simulink model "Consensus_Swarm"  (R2023b)
settings: Solver=ode3  StartTime=0.0  StopTime=inf  FixedStep=0.001  RelTol=1e-3
values from neighbouring files (symbols this model uses):
  g = 9.8    [Parameters.m]
  Ic = [2 0 0; 0 2 0; 0 0 4]    [Parameters.m]
  m = 1    [Parameters.m]
  M_RB = [eye(3), zeros(3); zeros(3), I]    [Parameters.m]
  SAVE_SPACE = 5    [Parameters.m]
  STEP_SIZE = 1    [Parameters.m]
libraries: simulink_extras x36, slpidlib x36, aerolibutil x12, vrlib x7
(part 2 of 6)

== system Consensus_Swarm/Formatting/Euler to VR5 ==
  Euler Angles : Inport
  Axis Angle Vector : Subsystem
  Mux : Mux  Inputs=2
  Mux1 : Mux  Inputs=2
  Mux2 : Mux  Inputs=2
  Quaternion Multiplication (Pitch & Yaw) : aerolibutil/Quaternion Multiplication
  Quaternion Multiplication (Roll) : aerolibutil/Quaternion Multiplication
  Quaternion Normalization : Subsystem
  Quaternion Normalization1 : Subsystem
  Quaternion Normalization2 : Subsystem
  Selector : Selector  InputPortWidth=3  IndexOptions=Index vector (dialog)  Indices=[3]  OutputSizes=1
  Selector1 : Selector  InputPortWidth=3  IndexOptions=Index vector (dialog)  Indices=[2]  OutputSizes=1
  Selector2 : Selector  InputPortWidth=3  IndexOptions=Index vector (dialog)  Indices=[1]  OutputSizes=1
  Vr Pitch Axes : Constant  Value=[0 0 1]
  Vr Roll Axes : Constant  Value=[1 0 0]
  Vr Yaw Axes : Constant  Value=[0 -1 0]
  Axis Angle : Outport  VectorParamsAs1DForOutWhenUnconnected=off
  wires:
  Quaternion Multiplication (Roll)/1 -> Axis Angle Vector/1(e0)
  Axis Angle Vector/1(e0_norm) -> Axis Angle/1
  Quaternion Normalization/1(e0_norm) -> Quaternion Multiplication (Roll)/2
  Quaternion Normalization2/1(e0_norm) -> Quaternion Multiplication (Pitch & Yaw)/1
  Quaternion Normalization1/1(e0_norm) -> Quaternion Multiplication (Pitch & Yaw)/2
  Mux2/1 -> Quaternion Normalization2/1(e0)
  Mux1/1 -> Quaternion Normalization1/1(e0)
  Mux/1 -> Quaternion Normalization/1(e0)
  Selector/1 -> Mux2/1
  Vr Yaw Axes/1 -> Mux2/2
  Selector1/1 -> Mux1/1
  Vr Pitch Axes/1 -> Mux1/2
  Selector2/1 -> Mux/1
  Vr Roll Axes/1 -> Mux/2
  Euler Angles/1 -> Selector2/1, Selector1/1, Selector/1
  Quaternion Multiplication (Pitch & Yaw)/1 -> Quaternion Multiplication (Roll)/1

== system Consensus_Swarm/Formatting/Subsystem ==
  Propeller velocities : Inport
  Bias : Bias  Bias=.1  SaturateOnIntegerOverflow=off
  Bias1 : Bias  Bias=-.3  SaturateOnIntegerOverflow=off
  Bias2 : Bias  Bias=.5  SaturateOnIntegerOverflow=off
  Bias3 : Bias  Bias=.7  SaturateOnIntegerOverflow=off
  Constant : Constant  Value=[0 1 0]
  Data Type Conversion : DataTypeConversion  OutDataTypeStr=double  SaturateOnIntegerOverflow=off  RndMeth=Floor
  Demux : Demux
  Gain : Gain  Gain=1.38408
  Integrator : Integrator  InitialCondition=[.1 ; .2 ;-.3 ;-.4]  WrapState=on  WrappedStateUpperValue=2*pi  WrappedStateLowerValue=-2*pi
  Mux{,1..3} (4 alike) : Mux  Inputs=2
  Rate Transition2 : RateTransition
  Position Blade1 : Outport  VectorParamsAs1DForOutWhenUnconnected=off
  Position Blade 2 : Outport  Port=2  VectorParamsAs1DForOutWhenUnconnected=off
  Position Blade 3 : Outport  Port=3  VectorParamsAs1DForOutWhenUnconnected=off
  Position Blade 4 : Outport  Port=4  VectorParamsAs1DForOutWhenUnconnected=off
  wires:
  Bias3/1 -> Mux3/2
  Mux3/1 -> Position Blade 4/1
  Bias1/1 -> Mux1/2
  Bias2/1 -> Mux2/2
  Demux/2 -> Bias1/1
  Constant/1 -> Mux3/1, Mux2/1, Mux1/1, Mux/1
  Mux1/1 -> Position Blade 2/1
  Mux2/1 -> Position Blade 3/1
  Integrator/1 -> Rate Transition2/1
  Mux/1 -> Position Blade1/1
  Demux/3 -> Bias2/1
  Bias/1 -> Mux/2
  Propeller velocities/1 -> Data Type Conversion/1
  Demux/4 -> Bias3/1
  Rate Transition2/1 -> Demux/1
  Demux/1 -> Bias/1
  Data Type Conversion/1 -> Gain/1
  Gain/1 -> Integrator/1

== system Consensus_Swarm/Subsystem/LIDER ==
  (x,y,z,psi) : Inport
  GamePad : Inport  Port=2
  Constant2 : Constant  Value=[0;-0;-40]  VectorParams1D=off
  Degrees to Radians : simulink_extras/Transformations/Degrees to Radians
  Demux1 : Demux  Outputs=6
  Flight Control System : Subsystem
      settings: PortSchema="{\"entries\":[{\"content\":{\"sides\":[{\"content\":{\"connectorIds\":[\"In1\",\"In2\"]},\"type\":\"ConnectorPlacement.EquallySpacedRectSide\",\"uuid\":\"8ffec179-99fb-4b4c-a09d-a73fa0154dea\"},{\"content\":{\"connectorIds\":[\"Out1\"],\"side\":\"RIGHT\"},\"type\":\"ConnectorPlacement.EquallySpacedRectSide\",\"uuid\":\"b9ff487d-1da1-449a-81c9-f1838b0d3727\"},{\"content\":{\"connectorIds\":[\"In3\"],\"side\":\"TOP\"},\"type\":\"ConnectorPlacement.EquallySpacedRectSide\",\"uuid\":\"1948ac9a-8b1f-4a62-833b-18e2b106d39d\"}]},\"type\":\"ConnectorPlacement.EquallySpacedConnector\",\"uuid\":\"fea635f7-9753-4696-bad7-e2485c1b5acc\"}],\"packageUris\":[\"http://schema.mathworks.com/mf0/Connector/R2020b\"],\"version\":\"1.0\"}"
  Manual Switch : ManualSwitch  CurrentSetting=0
  Manual Switch1 : ManualSwitch  CurrentSetting=0
  Mux : Mux  Inputs=2
  OL inputs : Constant  Value=[0;0;0;0]  VectorParams1D=off
  Position refs (x,y,z,psi) : Constant  Value=[20;20;-17;-45]  VectorParams1D=off
  Quadcopter model : Subsystem
      settings: PortSchema="{\"entries\":[{\"content\":{\"sides\":[{\"content\":{\"connectorIds\":[\"In1\"]},\"type\":\"ConnectorPlacement.EquallySpacedRectSide\",\"uuid\":\"c5c2dfb8-9ff8-4aa4-96a6-7fa0d886c51f\"},{\"content\":{\"connectorIds\":[\"Out1\"],\"side\":\"RIGHT\"},\"type\":\"ConnectorPlacement.EquallySpacedRectSide\",\"uuid\":\"2d7c7d5c-4ac5-4ebd-b09f-6a78733e851d\"},{\"content\":{\"connectorIds\":[\"In2\"],\"side\":\"TOP\"},\"type\":\"ConnectorPlacement.EquallySpacedRectSide\",\"uuid\":\"cf3a786d-06ed-46d4-985b-5c210afb13ec\"}]},\"type\":\"ConnectorPlacement.EquallySpacedConnector\",\"uuid\":\"cd57f0e6-7b9c-4392-8478-6e8af8e2560e\"}],\"packageUris\":[\"http://schema.mathworks.com/mf0/Connector/R2020b\"],\"version\":\"1.0\"}"
  Radians to Degrees : simulink_extras/Transformations/Radians to Degrees
  Radians to Degrees1 : simulink_extras/Transformations/Radians to Degrees
  Radians to Degrees2 : simulink_extras/Transformations/Radians to Degrees
  p(0) : Constant  Value=[100;100;-100]  VectorParams1D=off
  phi(t) : Scope
  psi(t) : Scope
  theta(t) : Scope
  x(t) : Scope
  y(t) : Scope
  z(t) : Scope
  Eta : Outport
  wires:
  Radians to Degrees2/1 -> psi(t)/1
  Quadcopter model/1(eta) -> Eta/1, Demux1/1, Flight Control System/2(eta)
  OL inputs/1 -> Manual Switch/1
  Demux1/2 -> y(t)/1
  Constant2/1 -> Degrees to Radians/1
  p(0)/1 -> Mux/1
  Degrees to Radians/1 -> Mux/2
  Demux1/1 -> x(t)/1
  Radians to Degrees/1 -> phi(t)/1
  Demux1/4 -> Radians to Degrees/1
  Manual Switch1/1 -> Flight Control System/1(Pos. refs)
  Radians to Degrees1/1 -> theta(t)/1
  Demux1/3 -> z(t)/1
  Demux1/6 -> Radians to Degrees2/1
  Manual Switch/1 -> Quadcopter model/1(Fz,mx,my,mz)
  Demux1/5 -> Radians to Degrees1/1
  Position refs (x,y,z,psi)/1 -> Manual Switch1/1
  Flight Control System/1(Fz,mx,my,mz) -> Manual Switch/2
  Mux/1 -> Quadcopter model/2(init. cond.)
  (x,y,z,psi)/1 -> Manual Switch1/2
  GamePad/1 -> Flight Control System/3(gamepad input)

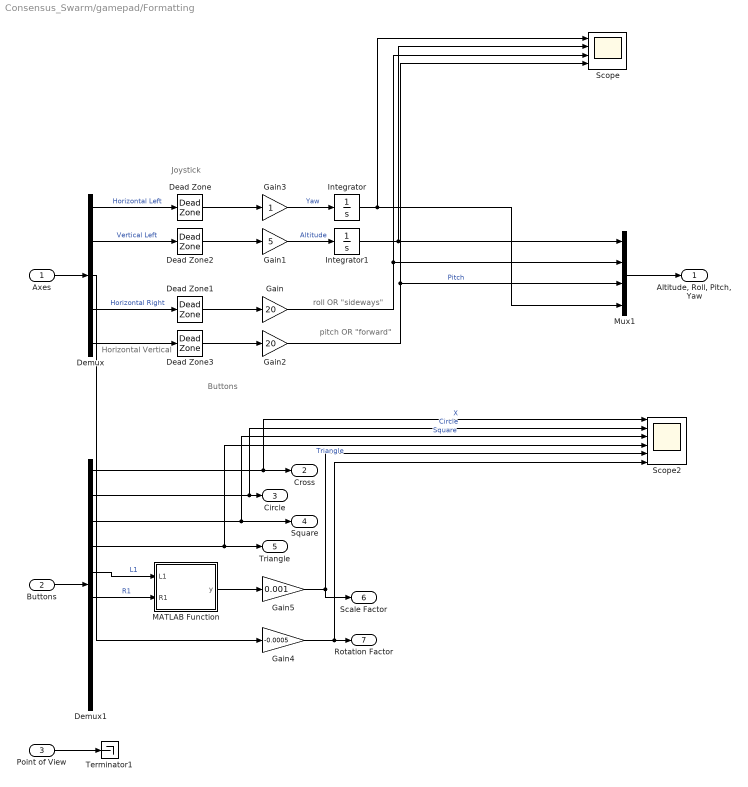
== system Consensus_Swarm/gamepad/Formatting ==
  note: Joystick
  note: Horizontal Vertical
  note: roll OR "sideways"
  note: pitch OR "forward"
  note: Buttons
  Axes : Inport
  Buttons : Inport  Port=2
  Point of View : Inport  Port=3
  Dead Zone{,1..3} (4 alike) : DeadZone  LowerValue=-0.2  UpperValue=0.2
  Demux : Demux  Outputs=5
  Demux1 : Demux  Outputs=10
  Gain : Gain  Gain=20
  Gain1 : Gain  Gain=5
  Gain2 : Gain  Gain=20
  Gain3 : Gain
  Gain4 : Gain  Gain=-0.0005
  Gain5 : Gain  Gain=0.001
  Integrator : Integrator
  Integrator1 : Integrator
  MATLAB Function : MATLAB Function  TreatAsAtomicUnit=on
  Mux1 : Mux
  Scope : Scope  NumInputPorts=4
  Scope2 : Scope  NumInputPorts=6
  Terminator1 : Terminator
  "Altitude, Roll, Pitch, Yaw" : Outport
  Cross : Outport  Port=2
  Circle : Outport  Port=3
  Square : Outport  Port=4
  Triangle : Outport  Port=5
  Scale Factor : Outport  Port=6
  Rotation Factor : Outport  Port=7
  wires:
  Axes/1 -> Demux/1
  Demux/5 -> Dead Zone3/1
  Demux/4 -> Dead Zone1/1  "Horizontal Right"
  Demux/1 -> Dead Zone/1  "Horizontal Left"
  Dead Zone1/1 -> Gain/1
  Demux/2 -> Dead Zone2/1  "Vertical Left"
  Dead Zone2/1 -> Gain1/1
  Dead Zone/1 -> Gain3/1
  Point of View/1 -> Terminator1/1
  Dead Zone3/1 -> Gain2/1
  Gain2/1 -> Scope/4, Mux1/3  "Pitch"
  Gain3/1 -> Integrator/1  "Yaw"
  Gain1/1 -> Integrator1/1  "Altitude"
  Buttons/1 -> Demux1/1
  Demux1/1 -> Scope2/1, Cross/1  "X"
  Demux1/2 -> Scope2/2, Circle/1  "Circle"
  Demux1/3 -> Square/1, Scope2/3  "Square"
  Demux1/4 -> Scope2/4, Triangle/1  "Triangle"
  Demux/3 -> Gain4/1
  Demux1/5 -> MATLAB Function/1(L1)  "L1"
  Gain5/1 -> Scope2/5, Scale Factor/1
  Gain4/1 -> Scope2/6, Rotation Factor/1
  Demux1/6 -> MATLAB Function/2(R1)  "R1"
  MATLAB Function/1(y) -> Gain5/1
  Mux1/1 -> "Altitude, Roll, Pitch, Yaw"/1
  Integrator/1 -> Scope/1, Mux1/4
  Integrator1/1 -> Scope/2, Mux1/1
  Gain/1 -> Scope/3, Mux1/2

== system Consensus_Swarm/FOLLOWER 1/Agent Model/Flight Control System ==
  Pos. refs : Inport
  eta : Inport  Port=2
  gamepad input : Inport  Port=3
  Inner-loop PID controllers : Subsystem
  Manual Switch : ManualSwitch  CurrentSetting=0
  Outer loop position control : Subsystem
  m_y(t) : Scope
  Fz,mx,my,mz : Outport
  wires:
  Inner-loop PID controllers/1(Fz,mx,my,mz) -> Fz,mx,my,mz/1
  Manual Switch/1 -> Inner-loop PID controllers/1(desired z,phi,theta,psi)
  eta/1 -> Outer loop position control/2(eta), Inner-loop PID controllers/2(eta)
  Pos. refs/1 -> Outer loop position control/1(Pos. refs)
  Outer loop position control/1(desired z,phi,theta,psi) -> Manual Switch/2
  gamepad input/1 -> Manual Switch/1

== system Consensus_Swarm/FOLLOWER 1/Agent Model/Quadcopter model ==
  note: $\eta$
  Fz,mx,my,mz : Inport
  init. cond. : Inport  Port=2
  Demux1 : Demux  Outputs=6
  Ground : Ground
  Ground1 : Ground
  Kinematics : Subsystem
  Mux1 : Mux  Inputs=3
  Rigid-body dynamics : Subsystem
  gravity : Subsystem
  u : Scope
  eta : Outport
  wires:
  Fz,mx,my,mz/1 -> Mux1/3
  Ground/1 -> Mux1/2
  Ground1/1 -> Mux1/1
  Kinematics/1(R_be) -> gravity/1(R_be)
  Kinematics/2(eta) -> eta/1
  gravity/1(tau_g) -> Rigid-body dynamics/1(tau_g)
  Mux1/1 -> Rigid-body dynamics/2(tau_p)
  Rigid-body dynamics/1(nu) -> Demux1/1, Kinematics/1(nu)
  init. cond./1 -> Kinematics/2(init. cond.)
  Demux1/1 -> u/1

== system Consensus_Swarm/FOLLOWER 1/Agent Model/gamepad ==
  Formatting : Subsystem
  Gamepad : vrlib/Joystick Input  joyid=1  adjustports=on  forcefeed=off
  gamepad input : Outport
  wires:
  Formatting/1(gamepad input) -> gamepad input/1
  Gamepad/2 -> Formatting/2(Buttons)
  Gamepad/1 -> Formatting/1(Axes)
  Gamepad/3 -> Formatting/3(Point of View)

== system Consensus_Swarm/FOLLOWER 2/Agent Model/Flight Control System ==
  Pos. refs : Inport
  eta : Inport  Port=2
  gamepad input : Inport  Port=3
  Inner-loop PID controllers : Subsystem
  Manual Switch : ManualSwitch  CurrentSetting=0
  Outer loop position control : Subsystem
  m_y(t) : Scope
  Fz,mx,my,mz : Outport
  wires:
  Inner-loop PID controllers/1(Fz,mx,my,mz) -> Fz,mx,my,mz/1
  Manual Switch/1 -> Inner-loop PID controllers/1(desired z,phi,theta,psi)
  eta/1 -> Outer loop position control/2(eta), Inner-loop PID controllers/2(eta)
  Pos. refs/1 -> Outer loop position control/1(Pos. refs)
  Outer loop position control/1(desired z,phi,theta,psi) -> Manual Switch/2
  gamepad input/1 -> Manual Switch/1

== system Consensus_Swarm/FOLLOWER 2/Agent Model/Quadcopter model ==
  note: $\eta$
  Fz,mx,my,mz : Inport
  init. cond. : Inport  Port=2
  Demux1 : Demux  Outputs=6
  Ground : Ground
  Ground1 : Ground
  Kinematics : Subsystem
  Mux1 : Mux  Inputs=3
  Rigid-body dynamics : Subsystem
  gravity : Subsystem
  u : Scope
  eta : Outport
  wires:
  Fz,mx,my,mz/1 -> Mux1/3
  Ground/1 -> Mux1/2
  Ground1/1 -> Mux1/1
  Kinematics/1(R_be) -> gravity/1(R_be)
  Kinematics/2(eta) -> eta/1
  gravity/1(tau_g) -> Rigid-body dynamics/1(tau_g)
  Mux1/1 -> Rigid-body dynamics/2(tau_p)
  Rigid-body dynamics/1(nu) -> Demux1/1, Kinematics/1(nu)
  init. cond./1 -> Kinematics/2(init. cond.)
  Demux1/1 -> u/1

== system Consensus_Swarm/FOLLOWER 2/Agent Model/gamepad ==
  Formatting : Subsystem
  Gamepad : vrlib/Joystick Input  joyid=1  adjustports=on  forcefeed=off
  gamepad input : Outport
  wires:
  Formatting/1(gamepad input) -> gamepad input/1
  Gamepad/2 -> Formatting/2(Buttons)
  Gamepad/1 -> Formatting/1(Axes)
  Gamepad/3 -> Formatting/3(Point of View)

== system Consensus_Swarm/FOLLOWER 3/Agent Model/Flight Control System ==
  Pos. refs : Inport
  eta : Inport  Port=2
  gamepad input : Inport  Port=3
  Inner-loop PID controllers : Subsystem
  Manual Switch : ManualSwitch  CurrentSetting=0
  Outer loop position control : Subsystem
  m_y(t) : Scope
  Fz,mx,my,mz : Outport
  wires:
  Inner-loop PID controllers/1(Fz,mx,my,mz) -> Fz,mx,my,mz/1
  Manual Switch/1 -> Inner-loop PID controllers/1(desired z,phi,theta,psi)
  eta/1 -> Outer loop position control/2(eta), Inner-loop PID controllers/2(eta)
  Pos. refs/1 -> Outer loop position control/1(Pos. refs)
  Outer loop position control/1(desired z,phi,theta,psi) -> Manual Switch/2
  gamepad input/1 -> Manual Switch/1

== system Consensus_Swarm/FOLLOWER 3/Agent Model/Quadcopter model ==
  note: $\eta$
  Fz,mx,my,mz : Inport
  init. cond. : Inport  Port=2
  Demux1 : Demux  Outputs=6
  Ground : Ground
  Ground1 : Ground
  Kinematics : Subsystem
  Mux1 : Mux  Inputs=3
  Rigid-body dynamics : Subsystem
  gravity : Subsystem
  u : Scope
  eta : Outport
  wires:
  Fz,mx,my,mz/1 -> Mux1/3
  Ground/1 -> Mux1/2
  Ground1/1 -> Mux1/1
  Kinematics/1(R_be) -> gravity/1(R_be)
  Kinematics/2(eta) -> eta/1
  gravity/1(tau_g) -> Rigid-body dynamics/1(tau_g)
  Mux1/1 -> Rigid-body dynamics/2(tau_p)
  Rigid-body dynamics/1(nu) -> Demux1/1, Kinematics/1(nu)
  init. cond./1 -> Kinematics/2(init. cond.)
  Demux1/1 -> u/1

== system Consensus_Swarm/FOLLOWER 3/Agent Model/gamepad ==
  Formatting : Subsystem
  Gamepad : vrlib/Joystick Input  joyid=1  adjustports=on  forcefeed=off
  gamepad input : Outport
  wires:
  Formatting/1(gamepad input) -> gamepad input/1
  Gamepad/2 -> Formatting/2(Buttons)
  Gamepad/1 -> Formatting/1(Axes)
  Gamepad/3 -> Formatting/3(Point of View)

== system Consensus_Swarm/FOLLOWER 4/Agent Model/Flight Control System ==
  Pos. refs : Inport
  eta : Inport  Port=2
  gamepad input : Inport  Port=3
  Inner-loop PID controllers : Subsystem
  Manual Switch : ManualSwitch  CurrentSetting=0
  Outer loop position control : Subsystem
  m_y(t) : Scope
  Fz,mx,my,mz : Outport
  wires:
  Inner-loop PID controllers/1(Fz,mx,my,mz) -> Fz,mx,my,mz/1
  Manual Switch/1 -> Inner-loop PID controllers/1(desired z,phi,theta,psi)
  eta/1 -> Outer loop position control/2(eta), Inner-loop PID controllers/2(eta)
  Pos. refs/1 -> Outer loop position control/1(Pos. refs)
  Outer loop position control/1(desired z,phi,theta,psi) -> Manual Switch/2
  gamepad input/1 -> Manual Switch/1

== system Consensus_Swarm/FOLLOWER 4/Agent Model/Quadcopter model ==
  note: $\eta$
  Fz,mx,my,mz : Inport
  init. cond. : Inport  Port=2
  Demux1 : Demux  Outputs=6
  Ground : Ground
  Ground1 : Ground
  Kinematics : Subsystem
  Mux1 : Mux  Inputs=3
  Rigid-body dynamics : Subsystem
  gravity : Subsystem
  u : Scope
  eta : Outport
  wires:
  Fz,mx,my,mz/1 -> Mux1/3
  Ground/1 -> Mux1/2
  Ground1/1 -> Mux1/1
  Kinematics/1(R_be) -> gravity/1(R_be)
  Kinematics/2(eta) -> eta/1
  gravity/1(tau_g) -> Rigid-body dynamics/1(tau_g)
  Mux1/1 -> Rigid-body dynamics/2(tau_p)
  Rigid-body dynamics/1(nu) -> Demux1/1, Kinematics/1(nu)
  init. cond./1 -> Kinematics/2(init. cond.)
  Demux1/1 -> u/1

== system Consensus_Swarm/FOLLOWER 4/Agent Model/gamepad ==
  Formatting : Subsystem
  Gamepad : vrlib/Joystick Input  joyid=1  adjustports=on  forcefeed=off
  gamepad input : Outport
  wires:
  Formatting/1(gamepad input) -> gamepad input/1
  Gamepad/2 -> Formatting/2(Buttons)
  Gamepad/1 -> Formatting/1(Axes)
  Gamepad/3 -> Formatting/3(Point of View)

== system Consensus_Swarm/FOLLOWER 5/Agent Model/Flight Control System ==
  Pos. refs : Inport
  eta : Inport  Port=2
  gamepad input : Inport  Port=3
  Inner-loop PID controllers : Subsystem
  Manual Switch : ManualSwitch  CurrentSetting=0
  Outer loop position control : Subsystem
  m_y(t) : Scope
  Fz,mx,my,mz : Outport
  wires:
  Inner-loop PID controllers/1(Fz,mx,my,mz) -> Fz,mx,my,mz/1
  Manual Switch/1 -> Inner-loop PID controllers/1(desired z,phi,theta,psi)
  eta/1 -> Outer loop position control/2(eta), Inner-loop PID controllers/2(eta)
  Pos. refs/1 -> Outer loop position control/1(Pos. refs)
  Outer loop position control/1(desired z,phi,theta,psi) -> Manual Switch/2
  gamepad input/1 -> Manual Switch/1

== system Consensus_Swarm/FOLLOWER 5/Agent Model/Quadcopter model ==
  note: $\eta$
  Fz,mx,my,mz : Inport
  init. cond. : Inport  Port=2
  Demux1 : Demux  Outputs=6
  Ground : Ground
  Ground1 : Ground
  Kinematics : Subsystem
  Mux1 : Mux  Inputs=3
  Rigid-body dynamics : Subsystem
  gravity : Subsystem
  u : Scope
  eta : Outport
  wires:
  Fz,mx,my,mz/1 -> Mux1/3
  Ground/1 -> Mux1/2
  Ground1/1 -> Mux1/1
  Kinematics/1(R_be) -> gravity/1(R_be)
  Kinematics/2(eta) -> eta/1
  gravity/1(tau_g) -> Rigid-body dynamics/1(tau_g)
  Mux1/1 -> Rigid-body dynamics/2(tau_p)
  Rigid-body dynamics/1(nu) -> Demux1/1, Kinematics/1(nu)
  init. cond./1 -> Kinematics/2(init. cond.)
  Demux1/1 -> u/1

== system Consensus_Swarm/FOLLOWER 5/Agent Model/gamepad ==
  Formatting : Subsystem
  Gamepad : vrlib/Joystick Input  joyid=1  adjustports=on  forcefeed=off
  gamepad input : Outport
  wires:
  Formatting/1(gamepad input) -> gamepad input/1
  Gamepad/2 -> Formatting/2(Buttons)
  Gamepad/1 -> Formatting/1(Axes)
  Gamepad/3 -> Formatting/3(Point of View)

== system Consensus_Swarm/Formatting/Euler to VR/Axis Angle Vector ==
  e0 : Inport
  2 : Gain  Gain=2  SaturateOnIntegerOverflow=on  OutDataTypeStr=Inherit: Same as input  ParamDataTypeStr=Inherit: Same as input
  Constant : Constant  Value=1e-6
  Demux : Demux  Outputs=[1 3 ]
      settings: DisplayOption=none
  Mux : Mux  Inputs=2
  Product : Product  Inputs=*/  InputSameDT=on  SaturateOnIntegerOverflow=on  OutDataTypeStr=Inherit: Same as first input
  Switch : Switch  Criteria=u2 ~= 0  SaturateOnIntegerOverflow=off  InputSameDT=off
  Trigonometric Function : Trigonometry
  Trigonometric Function2 : Trigonometry  Operator=acos
  e0_norm : Outport  VectorParamsAs1DForOutWhenUnconnected=off
  wires:
  Demux/1 -> Trigonometric Function2/1
  Demux/2 -> Product/1
  Mux/1 -> e0_norm/1
  Product/1 -> Mux/1
  2/1 -> Mux/2
  Trigonometric Function/1 -> Switch/1, Switch/2
  Trigonometric Function2/1 -> Trigonometric Function/1, 2/1
  e0/1 -> Demux/1
  Constant/1 -> Switch/3
  Switch/1 -> Product/2

== system Consensus_Swarm/Formatting/Euler to VR/Quaternion Normalization ==
  e0 : Inport
  1/2 : Gain  Gain=1/2  SaturateOnIntegerOverflow=on  OutDataTypeStr=Inherit: Same as input  ParamDataTypeStr=Inherit: Same as input
  Demux : Demux  Outputs=[1 3]
      settings: DisplayOption=none
  Mux : Mux  Inputs=2
  Product : Product  InputSameDT=on  SaturateOnIntegerOverflow=on  OutDataTypeStr=Inherit: Same as first input
  Trigonometric Function : Trigonometry
  Trigonometric Function1 : Trigonometry  Operator=cos
  e0_norm : Outport  VectorParamsAs1DForOutWhenUnconnected=off
  wires:
  Trigonometric Function1/1 -> Mux/1
  Demux/2 -> Product/2
  Demux/1 -> 1/2/1
  Mux/1 -> e0_norm/1
  Product/1 -> Mux/2
  Trigonometric Function/1 -> Product/1
  1/2/1 -> Trigonometric Function1/1, Trigonometric Function/1
  e0/1 -> Demux/1

== system Consensus_Swarm/Formatting/Euler to VR/Quaternion Normalization1 ==
  e0 : Inport
  1/2 : Gain  Gain=1/2  SaturateOnIntegerOverflow=on  OutDataTypeStr=Inherit: Same as input  ParamDataTypeStr=Inherit: Same as input
  Demux : Demux  Outputs=[1 3]
      settings: DisplayOption=none
  Mux : Mux  Inputs=2
  Product : Product  InputSameDT=on  SaturateOnIntegerOverflow=on  OutDataTypeStr=Inherit: Same as first input
  Trigonometric Function : Trigonometry
  Trigonometric Function1 : Trigonometry  Operator=cos
  e0_norm : Outport  VectorParamsAs1DForOutWhenUnconnected=off
  wires:
  e0/1 -> Demux/1
  1/2/1 -> Trigonometric Function/1, Trigonometric Function1/1
  Trigonometric Function/1 -> Product/1
  Product/1 -> Mux/2
  Mux/1 -> e0_norm/1
  Demux/1 -> 1/2/1
  Demux/2 -> Product/2
  Trigonometric Function1/1 -> Mux/1

== system Consensus_Swarm/Formatting/Euler to VR/Quaternion Normalization2 ==
  e0 : Inport
  1/2 : Gain  Gain=1/2  SaturateOnIntegerOverflow=on  OutDataTypeStr=Inherit: Same as input  ParamDataTypeStr=Inherit: Same as input
  Demux : Demux  Outputs=[1 3]
      settings: DisplayOption=none
  Mux : Mux  Inputs=2
  Product : Product  InputSameDT=on  SaturateOnIntegerOverflow=on  OutDataTypeStr=Inherit: Same as first input
  Trigonometric Function : Trigonometry
  Trigonometric Function1 : Trigonometry  Operator=cos
  e0_norm : Outport  VectorParamsAs1DForOutWhenUnconnected=off
  wires:
  Trigonometric Function1/1 -> Mux/1
  Demux/2 -> Product/2
  Demux/1 -> 1/2/1
  Mux/1 -> e0_norm/1
  Product/1 -> Mux/2
  Trigonometric Function/1 -> Product/1
  1/2/1 -> Trigonometric Function1/1, Trigonometric Function/1
  e0/1 -> Demux/1

== system Consensus_Swarm/Formatting/Euler to VR1/Axis Angle Vector ==
  e0 : Inport
  2 : Gain  Gain=2  SaturateOnIntegerOverflow=on  OutDataTypeStr=Inherit: Same as input  ParamDataTypeStr=Inherit: Same as input
  Constant : Constant  Value=1e-6
  Demux : Demux  Outputs=[1 3 ]
      settings: DisplayOption=none
  Mux : Mux  Inputs=2
  Product : Product  Inputs=*/  InputSameDT=on  SaturateOnIntegerOverflow=on  OutDataTypeStr=Inherit: Same as first input
  Switch : Switch  Criteria=u2 ~= 0  SaturateOnIntegerOverflow=off  InputSameDT=off
  Trigonometric Function : Trigonometry
  Trigonometric Function2 : Trigonometry  Operator=acos
  e0_norm : Outport  VectorParamsAs1DForOutWhenUnconnected=off
  wires:
  Demux/1 -> Trigonometric Function2/1
  Demux/2 -> Product/1
  Mux/1 -> e0_norm/1
  Product/1 -> Mux/1
  2/1 -> Mux/2
  Trigonometric Function/1 -> Switch/1, Switch/2
  Trigonometric Function2/1 -> Trigonometric Function/1, 2/1
  e0/1 -> Demux/1
  Constant/1 -> Switch/3
  Switch/1 -> Product/2

== system Consensus_Swarm/Formatting/Euler to VR1/Quaternion Normalization ==
  e0 : Inport
  1/2 : Gain  Gain=1/2  SaturateOnIntegerOverflow=on  OutDataTypeStr=Inherit: Same as input  ParamDataTypeStr=Inherit: Same as input
  Demux : Demux  Outputs=[1 3]
      settings: DisplayOption=none
  Mux : Mux  Inputs=2
  Product : Product  InputSameDT=on  SaturateOnIntegerOverflow=on  OutDataTypeStr=Inherit: Same as first input
  Trigonometric Function : Trigonometry
  Trigonometric Function1 : Trigonometry  Operator=cos
  e0_norm : Outport  VectorParamsAs1DForOutWhenUnconnected=off
  wires:
  Trigonometric Function1/1 -> Mux/1
  Demux/2 -> Product/2
  Demux/1 -> 1/2/1
  Mux/1 -> e0_norm/1
  Product/1 -> Mux/2
  Trigonometric Function/1 -> Product/1
  1/2/1 -> Trigonometric Function1/1, Trigonometric Function/1
  e0/1 -> Demux/1

== system Consensus_Swarm/Formatting/Euler to VR1/Quaternion Normalization1 ==
  e0 : Inport
  1/2 : Gain  Gain=1/2  SaturateOnIntegerOverflow=on  OutDataTypeStr=Inherit: Same as input  ParamDataTypeStr=Inherit: Same as input
  Demux : Demux  Outputs=[1 3]
      settings: DisplayOption=none
  Mux : Mux  Inputs=2
  Product : Product  InputSameDT=on  SaturateOnIntegerOverflow=on  OutDataTypeStr=Inherit: Same as first input
  Trigonometric Function : Trigonometry
  Trigonometric Function1 : Trigonometry  Operator=cos
  e0_norm : Outport  VectorParamsAs1DForOutWhenUnconnected=off
  wires:
  e0/1 -> Demux/1
  1/2/1 -> Trigonometric Function/1, Trigonometric Function1/1
  Trigonometric Function/1 -> Product/1
  Product/1 -> Mux/2
  Mux/1 -> e0_norm/1
  Demux/1 -> 1/2/1
  Demux/2 -> Product/2
  Trigonometric Function1/1 -> Mux/1

== system Consensus_Swarm/Formatting/Euler to VR1/Quaternion Normalization2 ==
  e0 : Inport
  1/2 : Gain  Gain=1/2  SaturateOnIntegerOverflow=on  OutDataTypeStr=Inherit: Same as input  ParamDataTypeStr=Inherit: Same as input
  Demux : Demux  Outputs=[1 3]
      settings: DisplayOption=none
  Mux : Mux  Inputs=2
  Product : Product  InputSameDT=on  SaturateOnIntegerOverflow=on  OutDataTypeStr=Inherit: Same as first input
  Trigonometric Function : Trigonometry
  Trigonometric Function1 : Trigonometry  Operator=cos
  e0_norm : Outport  VectorParamsAs1DForOutWhenUnconnected=off
  wires:
  Trigonometric Function1/1 -> Mux/1
  Demux/2 -> Product/2
  Demux/1 -> 1/2/1
  Mux/1 -> e0_norm/1
  Product/1 -> Mux/2
  Trigonometric Function/1 -> Product/1
  1/2/1 -> Trigonometric Function1/1, Trigonometric Function/1
  e0/1 -> Demux/1

== system Consensus_Swarm/Formatting/Euler to VR2/Axis Angle Vector ==
  e0 : Inport
  2 : Gain  Gain=2  SaturateOnIntegerOverflow=on  OutDataTypeStr=Inherit: Same as input  ParamDataTypeStr=Inherit: Same as input
  Constant : Constant  Value=1e-6
  Demux : Demux  Outputs=[1 3 ]
      settings: DisplayOption=none
  Mux : Mux  Inputs=2
  Product : Product  Inputs=*/  InputSameDT=on  SaturateOnIntegerOverflow=on  OutDataTypeStr=Inherit: Same as first input
  Switch : Switch  Criteria=u2 ~= 0  SaturateOnIntegerOverflow=off  InputSameDT=off
  Trigonometric Function : Trigonometry
  Trigonometric Function2 : Trigonometry  Operator=acos
  e0_norm : Outport  VectorParamsAs1DForOutWhenUnconnected=off
  wires:
  Demux/1 -> Trigonometric Function2/1
  Demux/2 -> Product/1
  Mux/1 -> e0_norm/1
  Product/1 -> Mux/1
  2/1 -> Mux/2
  Trigonometric Function/1 -> Switch/1, Switch/2
  Trigonometric Function2/1 -> Trigonometric Function/1, 2/1
  e0/1 -> Demux/1
  Constant/1 -> Switch/3
  Switch/1 -> Product/2

== system Consensus_Swarm/Formatting/Euler to VR2/Quaternion Normalization ==
  e0 : Inport
  1/2 : Gain  Gain=1/2  SaturateOnIntegerOverflow=on  OutDataTypeStr=Inherit: Same as input  ParamDataTypeStr=Inherit: Same as input
  Demux : Demux  Outputs=[1 3]
      settings: DisplayOption=none
  Mux : Mux  Inputs=2
  Product : Product  InputSameDT=on  SaturateOnIntegerOverflow=on  OutDataTypeStr=Inherit: Same as first input
  Trigonometric Function : Trigonometry
  Trigonometric Function1 : Trigonometry  Operator=cos
  e0_norm : Outport  VectorParamsAs1DForOutWhenUnconnected=off
  wires:
  Trigonometric Function1/1 -> Mux/1
  Demux/2 -> Product/2
  Demux/1 -> 1/2/1
  Mux/1 -> e0_norm/1
  Product/1 -> Mux/2
  Trigonometric Function/1 -> Product/1
  1/2/1 -> Trigonometric Function1/1, Trigonometric Function/1
  e0/1 -> Demux/1

== system Consensus_Swarm/Formatting/Euler to VR2/Quaternion Normalization1 ==
  e0 : Inport
  1/2 : Gain  Gain=1/2  SaturateOnIntegerOverflow=on  OutDataTypeStr=Inherit: Same as input  ParamDataTypeStr=Inherit: Same as input
  Demux : Demux  Outputs=[1 3]
      settings: DisplayOption=none
  Mux : Mux  Inputs=2
  Product : Product  InputSameDT=on  SaturateOnIntegerOverflow=on  OutDataTypeStr=Inherit: Same as first input
  Trigonometric Function : Trigonometry
  Trigonometric Function1 : Trigonometry  Operator=cos
  e0_norm : Outport  VectorParamsAs1DForOutWhenUnconnected=off
  wires:
  e0/1 -> Demux/1
  1/2/1 -> Trigonometric Function/1, Trigonometric Function1/1
  Trigonometric Function/1 -> Product/1
  Product/1 -> Mux/2
  Mux/1 -> e0_norm/1
  Demux/1 -> 1/2/1
  Demux/2 -> Product/2
  Trigonometric Function1/1 -> Mux/1

== system Consensus_Swarm/Formatting/Euler to VR2/Quaternion Normalization2 ==
  e0 : Inport
  1/2 : Gain  Gain=1/2  SaturateOnIntegerOverflow=on  OutDataTypeStr=Inherit: Same as input  ParamDataTypeStr=Inherit: Same as input
  Demux : Demux  Outputs=[1 3]
      settings: DisplayOption=none
  Mux : Mux  Inputs=2
  Product : Product  InputSameDT=on  SaturateOnIntegerOverflow=on  OutDataTypeStr=Inherit: Same as first input
  Trigonometric Function : Trigonometry
  Trigonometric Function1 : Trigonometry  Operator=cos
  e0_norm : Outport  VectorParamsAs1DForOutWhenUnconnected=off
  wires:
  Trigonometric Function1/1 -> Mux/1
  Demux/2 -> Product/2
  Demux/1 -> 1/2/1
  Mux/1 -> e0_norm/1
  Product/1 -> Mux/2
  Trigonometric Function/1 -> Product/1
  1/2/1 -> Trigonometric Function1/1, Trigonometric Function/1
  e0/1 -> Demux/1

== system Consensus_Swarm/Formatting/Euler to VR3/Axis Angle Vector ==
  e0 : Inport
  2 : Gain  Gain=2  SaturateOnIntegerOverflow=on  OutDataTypeStr=Inherit: Same as input  ParamDataTypeStr=Inherit: Same as input
  Constant : Constant  Value=1e-6
  Demux : Demux  Outputs=[1 3 ]
      settings: DisplayOption=none
  Mux : Mux  Inputs=2
  Product : Product  Inputs=*/  InputSameDT=on  SaturateOnIntegerOverflow=on  OutDataTypeStr=Inherit: Same as first input
  Switch : Switch  Criteria=u2 ~= 0  SaturateOnIntegerOverflow=off  InputSameDT=off
  Trigonometric Function : Trigonometry
  Trigonometric Function2 : Trigonometry  Operator=acos
  e0_norm : Outport  VectorParamsAs1DForOutWhenUnconnected=off
  wires:
  Demux/1 -> Trigonometric Function2/1
  Demux/2 -> Product/1
  Mux/1 -> e0_norm/1
  Product/1 -> Mux/1
  2/1 -> Mux/2
  Trigonometric Function/1 -> Switch/1, Switch/2
  Trigonometric Function2/1 -> Trigonometric Function/1, 2/1
  e0/1 -> Demux/1
  Constant/1 -> Switch/3
  Switch/1 -> Product/2

== system Consensus_Swarm/Formatting/Euler to VR3/Quaternion Normalization ==
  e0 : Inport
  1/2 : Gain  Gain=1/2  SaturateOnIntegerOverflow=on  OutDataTypeStr=Inherit: Same as input  ParamDataTypeStr=Inherit: Same as input
  Demux : Demux  Outputs=[1 3]
      settings: DisplayOption=none
  Mux : Mux  Inputs=2
  Product : Product  InputSameDT=on  SaturateOnIntegerOverflow=on  OutDataTypeStr=Inherit: Same as first input
  Trigonometric Function : Trigonometry
  Trigonometric Function1 : Trigonometry  Operator=cos
  e0_norm : Outport  VectorParamsAs1DForOutWhenUnconnected=off
  wires:
  Trigonometric Function1/1 -> Mux/1
  Demux/2 -> Product/2
  Demux/1 -> 1/2/1
  Mux/1 -> e0_norm/1
  Product/1 -> Mux/2
  Trigonometric Function/1 -> Product/1
  1/2/1 -> Trigonometric Function1/1, Trigonometric Function/1
  e0/1 -> Demux/1

== system Consensus_Swarm/Formatting/Euler to VR3/Quaternion Normalization1 ==
  e0 : Inport
  1/2 : Gain  Gain=1/2  SaturateOnIntegerOverflow=on  OutDataTypeStr=Inherit: Same as input  ParamDataTypeStr=Inherit: Same as input
  Demux : Demux  Outputs=[1 3]
      settings: DisplayOption=none
  Mux : Mux  Inputs=2
  Product : Product  InputSameDT=on  SaturateOnIntegerOverflow=on  OutDataTypeStr=Inherit: Same as first input
  Trigonometric Function : Trigonometry
  Trigonometric Function1 : Trigonometry  Operator=cos
  e0_norm : Outport  VectorParamsAs1DForOutWhenUnconnected=off
  wires:
  e0/1 -> Demux/1
  1/2/1 -> Trigonometric Function/1, Trigonometric Function1/1
  Trigonometric Function/1 -> Product/1
  Product/1 -> Mux/2
  Mux/1 -> e0_norm/1
  Demux/1 -> 1/2/1
  Demux/2 -> Product/2
  Trigonometric Function1/1 -> Mux/1

== system Consensus_Swarm/Formatting/Euler to VR3/Quaternion Normalization2 ==
  e0 : Inport
  1/2 : Gain  Gain=1/2  SaturateOnIntegerOverflow=on  OutDataTypeStr=Inherit: Same as input  ParamDataTypeStr=Inherit: Same as input
  Demux : Demux  Outputs=[1 3]
      settings: DisplayOption=none
  Mux : Mux  Inputs=2
  Product : Product  InputSameDT=on  SaturateOnIntegerOverflow=on  OutDataTypeStr=Inherit: Same as first input
  Trigonometric Function : Trigonometry
  Trigonometric Function1 : Trigonometry  Operator=cos
  e0_norm : Outport  VectorParamsAs1DForOutWhenUnconnected=off
  wires:
  Trigonometric Function1/1 -> Mux/1
  Demux/2 -> Product/2
  Demux/1 -> 1/2/1
  Mux/1 -> e0_norm/1
  Product/1 -> Mux/2
  Trigonometric Function/1 -> Product/1
  1/2/1 -> Trigonometric Function1/1, Trigonometric Function/1
  e0/1 -> Demux/1

== system Consensus_Swarm/Formatting/Euler to VR4/Axis Angle Vector ==
  e0 : Inport
  2 : Gain  Gain=2  SaturateOnIntegerOverflow=on  OutDataTypeStr=Inherit: Same as input  ParamDataTypeStr=Inherit: Same as input
  Constant : Constant  Value=1e-6
  Demux : Demux  Outputs=[1 3 ]
      settings: DisplayOption=none
  Mux : Mux  Inputs=2
  Product : Product  Inputs=*/  InputSameDT=on  SaturateOnIntegerOverflow=on  OutDataTypeStr=Inherit: Same as first input
  Switch : Switch  Criteria=u2 ~= 0  SaturateOnIntegerOverflow=off  InputSameDT=off
  Trigonometric Function : Trigonometry
  Trigonometric Function2 : Trigonometry  Operator=acos
  e0_norm : Outport  VectorParamsAs1DForOutWhenUnconnected=off
  wires:
  Demux/1 -> Trigonometric Function2/1
  Demux/2 -> Product/1
  Mux/1 -> e0_norm/1
  Product/1 -> Mux/1
  2/1 -> Mux/2
  Trigonometric Function/1 -> Switch/1, Switch/2
  Trigonometric Function2/1 -> Trigonometric Function/1, 2/1
  e0/1 -> Demux/1
  Constant/1 -> Switch/3
  Switch/1 -> Product/2

== system Consensus_Swarm/Formatting/Euler to VR4/Quaternion Normalization ==
  e0 : Inport
  1/2 : Gain  Gain=1/2  SaturateOnIntegerOverflow=on  OutDataTypeStr=Inherit: Same as input  ParamDataTypeStr=Inherit: Same as input
  Demux : Demux  Outputs=[1 3]
      settings: DisplayOption=none
  Mux : Mux  Inputs=2
  Product : Product  InputSameDT=on  SaturateOnIntegerOverflow=on  OutDataTypeStr=Inherit: Same as first input
  Trigonometric Function : Trigonometry
  Trigonometric Function1 : Trigonometry  Operator=cos
  e0_norm : Outport  VectorParamsAs1DForOutWhenUnconnected=off
  wires:
  Trigonometric Function1/1 -> Mux/1
  Demux/2 -> Product/2
  Demux/1 -> 1/2/1
  Mux/1 -> e0_norm/1
  Product/1 -> Mux/2
  Trigonometric Function/1 -> Product/1
  1/2/1 -> Trigonometric Function1/1, Trigonometric Function/1
  e0/1 -> Demux/1

== system Consensus_Swarm/Formatting/Euler to VR4/Quaternion Normalization1 ==
  e0 : Inport
  1/2 : Gain  Gain=1/2  SaturateOnIntegerOverflow=on  OutDataTypeStr=Inherit: Same as input  ParamDataTypeStr=Inherit: Same as input
  Demux : Demux  Outputs=[1 3]
      settings: DisplayOption=none
  Mux : Mux  Inputs=2
  Product : Product  InputSameDT=on  SaturateOnIntegerOverflow=on  OutDataTypeStr=Inherit: Same as first input
  Trigonometric Function : Trigonometry
  Trigonometric Function1 : Trigonometry  Operator=cos
  e0_norm : Outport  VectorParamsAs1DForOutWhenUnconnected=off
  wires:
  e0/1 -> Demux/1
  1/2/1 -> Trigonometric Function/1, Trigonometric Function1/1
  Trigonometric Function/1 -> Product/1
  Product/1 -> Mux/2
  Mux/1 -> e0_norm/1
  Demux/1 -> 1/2/1
  Demux/2 -> Product/2
  Trigonometric Function1/1 -> Mux/1

== system Consensus_Swarm/Formatting/Euler to VR4/Quaternion Normalization2 ==
  e0 : Inport
  1/2 : Gain  Gain=1/2  SaturateOnIntegerOverflow=on  OutDataTypeStr=Inherit: Same as input  ParamDataTypeStr=Inherit: Same as input
  Demux : Demux  Outputs=[1 3]
      settings: DisplayOption=none
  Mux : Mux  Inputs=2
  Product : Product  InputSameDT=on  SaturateOnIntegerOverflow=on  OutDataTypeStr=Inherit: Same as first input
  Trigonometric Function : Trigonometry
  Trigonometric Function1 : Trigonometry  Operator=cos
  e0_norm : Outport  VectorParamsAs1DForOutWhenUnconnected=off
  wires:
  Trigonometric Function1/1 -> Mux/1
  Demux/2 -> Product/2
  Demux/1 -> 1/2/1
  Mux/1 -> e0_norm/1
  Product/1 -> Mux/2
  Trigonometric Function/1 -> Product/1
  1/2/1 -> Trigonometric Function1/1, Trigonometric Function/1
  e0/1 -> Demux/1

== system Consensus_Swarm/Formatting/Euler to VR5/Axis Angle Vector ==
  e0 : Inport
  2 : Gain  Gain=2  SaturateOnIntegerOverflow=on  OutDataTypeStr=Inherit: Same as input  ParamDataTypeStr=Inherit: Same as input
  Constant : Constant  Value=1e-6
  Demux : Demux  Outputs=[1 3 ]
      settings: DisplayOption=none
  Mux : Mux  Inputs=2
  Product : Product  Inputs=*/  InputSameDT=on  SaturateOnIntegerOverflow=on  OutDataTypeStr=Inherit: Same as first input
  Switch : Switch  Criteria=u2 ~= 0  SaturateOnIntegerOverflow=off  InputSameDT=off
  Trigonometric Function : Trigonometry
  Trigonometric Function2 : Trigonometry  Operator=acos
  e0_norm : Outport  VectorParamsAs1DForOutWhenUnconnected=off
  wires:
  Demux/1 -> Trigonometric Function2/1
  Demux/2 -> Product/1
  Mux/1 -> e0_norm/1
  Product/1 -> Mux/1
  2/1 -> Mux/2
  Trigonometric Function/1 -> Switch/1, Switch/2
  Trigonometric Function2/1 -> Trigonometric Function/1, 2/1
  e0/1 -> Demux/1
  Constant/1 -> Switch/3
  Switch/1 -> Product/2

== system Consensus_Swarm/Formatting/Euler to VR5/Quaternion Normalization ==
  e0 : Inport
  1/2 : Gain  Gain=1/2  SaturateOnIntegerOverflow=on  OutDataTypeStr=Inherit: Same as input  ParamDataTypeStr=Inherit: Same as input
  Demux : Demux  Outputs=[1 3]
      settings: DisplayOption=none
  Mux : Mux  Inputs=2
  Product : Product  InputSameDT=on  SaturateOnIntegerOverflow=on  OutDataTypeStr=Inherit: Same as first input
  Trigonometric Function : Trigonometry
  Trigonometric Function1 : Trigonometry  Operator=cos
  e0_norm : Outport  VectorParamsAs1DForOutWhenUnconnected=off
  wires:
  Trigonometric Function1/1 -> Mux/1
  Demux/2 -> Product/2
  Demux/1 -> 1/2/1
  Mux/1 -> e0_norm/1
  Product/1 -> Mux/2
  Trigonometric Function/1 -> Product/1
  1/2/1 -> Trigonometric Function1/1, Trigonometric Function/1
  e0/1 -> Demux/1

== system Consensus_Swarm/Formatting/Euler to VR5/Quaternion Normalization1 ==
  e0 : Inport
  1/2 : Gain  Gain=1/2  SaturateOnIntegerOverflow=on  OutDataTypeStr=Inherit: Same as input  ParamDataTypeStr=Inherit: Same as input
  Demux : Demux  Outputs=[1 3]
      settings: DisplayOption=none
  Mux : Mux  Inputs=2
  Product : Product  InputSameDT=on  SaturateOnIntegerOverflow=on  OutDataTypeStr=Inherit: Same as first input
  Trigonometric Function : Trigonometry
  Trigonometric Function1 : Trigonometry  Operator=cos
  e0_norm : Outport  VectorParamsAs1DForOutWhenUnconnected=off
  wires:
  e0/1 -> Demux/1
  1/2/1 -> Trigonometric Function/1, Trigonometric Function1/1
  Trigonometric Function/1 -> Product/1
  Product/1 -> Mux/2
  Mux/1 -> e0_norm/1
  Demux/1 -> 1/2/1
  Demux/2 -> Product/2
  Trigonometric Function1/1 -> Mux/1

== system Consensus_Swarm/Formatting/Euler to VR5/Quaternion Normalization2 ==
  e0 : Inport
  1/2 : Gain  Gain=1/2  SaturateOnIntegerOverflow=on  OutDataTypeStr=Inherit: Same as input  ParamDataTypeStr=Inherit: Same as input
  Demux : Demux  Outputs=[1 3]
      settings: DisplayOption=none
  Mux : Mux  Inputs=2
  Product : Product  InputSameDT=on  SaturateOnIntegerOverflow=on  OutDataTypeStr=Inherit: Same as first input
  Trigonometric Function : Trigonometry
  Trigonometric Function1 : Trigonometry  Operator=cos
  e0_norm : Outport  VectorParamsAs1DForOutWhenUnconnected=off
  wires:
  Trigonometric Function1/1 -> Mux/1
  Demux/2 -> Product/2
  Demux/1 -> 1/2/1
  Mux/1 -> e0_norm/1
  Product/1 -> Mux/2
  Trigonometric Function/1 -> Product/1
  1/2/1 -> Trigonometric Function1/1, Trigonometric Function/1
  e0/1 -> Demux/1

== system Consensus_Swarm/Subsystem/LIDER/Flight Control System ==
  Pos. refs : Inport
  eta : Inport  Port=2
  gamepad input : Inport  Port=3
  Inner-loop PID controllers : Subsystem
  Manual Switch : ManualSwitch
  Outer loop position control : Subsystem
  m_y(t) : Scope
  Fz,mx,my,mz : Outport
  wires:
  Inner-loop PID controllers/1(Fz,mx,my,mz) -> Fz,mx,my,mz/1
  Manual Switch/1 -> Inner-loop PID controllers/1(desired z,phi,theta,psi)
  eta/1 -> Outer loop position control/2(eta), Inner-loop PID controllers/2(eta)
  Pos. refs/1 -> Outer loop position control/1(Pos. refs)
  Outer loop position control/1(desired z,phi,theta,psi) -> Manual Switch/2
  gamepad input/1 -> Manual Switch/1

== system Consensus_Swarm/Subsystem/LIDER/Quadcopter model ==
  note: $\eta$
  Fz,mx,my,mz : Inport
  init. cond. : Inport  Port=2
  Demux1 : Demux  Outputs=6
  Ground : Ground
  Ground1 : Ground
  Kinematics : Subsystem
  Mux1 : Mux  Inputs=3
  Rigid-body dynamics : Subsystem
  gravity : Subsystem
  u : Scope
  eta : Outport
  wires:
  Fz,mx,my,mz/1 -> Mux1/3
  Ground/1 -> Mux1/2
  Ground1/1 -> Mux1/1
  Kinematics/1(R_be) -> gravity/1(R_be)
  Kinematics/2(eta) -> eta/1
  gravity/1(tau_g) -> Rigid-body dynamics/1(tau_g)
  Mux1/1 -> Rigid-body dynamics/2(tau_p)
  Rigid-body dynamics/1(nu) -> Demux1/1, Kinematics/1(nu)
  init. cond./1 -> Kinematics/2(init. cond.)
  Demux1/1 -> u/1
